simulink model "test"  (R2023b)
settings: Solver=VariableStepAuto  StartTime=0.0  StopTime=10.0  RelTol=1e-3
settings Model: Creator=yoany  LastModifiedBy=yoany

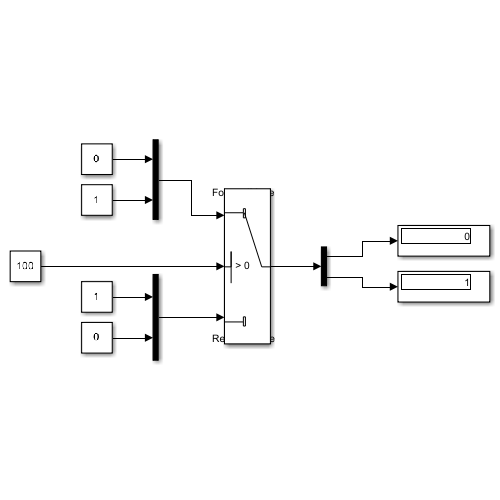
[thumbnail: Simulink's stored preview of the top-level diagram]
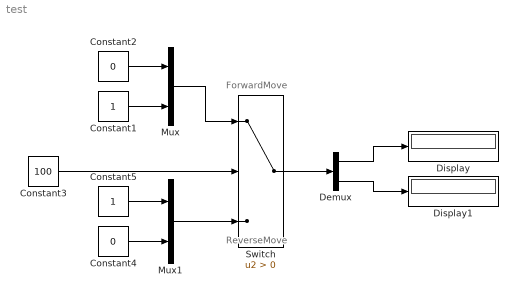
== system test ==
  note: ReverseMove
  note: ForwardMove
  Constant1 : Constant
  Constant2 : Constant  Value=0
  Constant3 : Constant  Value=100
  Constant4 : Constant  Value=0
  Constant5 : Constant
  Demux : Demux  Outputs=2
  Display : Display
  Display1 : Display
  Mux : Mux  Inputs=2
  Mux1 : Mux  Inputs=2
  Switch : Switch  Criteria=u2 > Threshold  SaturateOnIntegerOverflow=off  InputSameDT=off
  wires:
  Constant3/1 -> Switch/2
  Mux/1 -> Switch/1
  Constant2/1 -> Mux/1
  Constant1/1 -> Mux/2
  Mux1/1 -> Switch/3
  Constant4/1 -> Mux1/2
  Constant5/1 -> Mux1/1
  Switch/1 -> Demux/1
  Demux/1 -> Display/1
  Demux/2 -> Display1/1
